simulink library "CTRL_LO_ST1_YAWTRQLGT"  (R2023b)
settings: Solver=VariableStepAuto  StartTime=0.0  StopTime=10.0  RelTol=1e-3
settings Model: Creator=blatak  LastModifiedBy=blatak

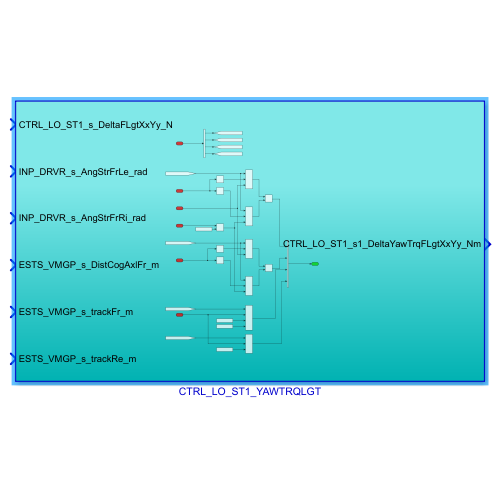
[thumbnail: Simulink's stored preview of the top-level diagram]
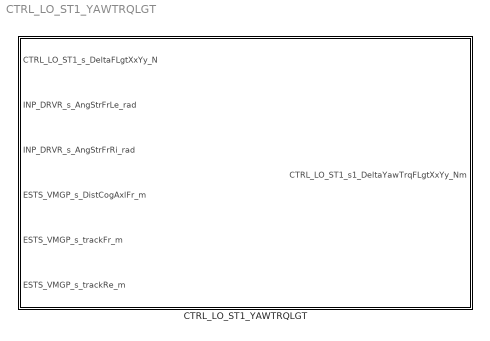
== system CTRL_LO_ST1_YAWTRQLGT ==
  CTRL_LO_ST1_YAWTRQLGT : Subsystem

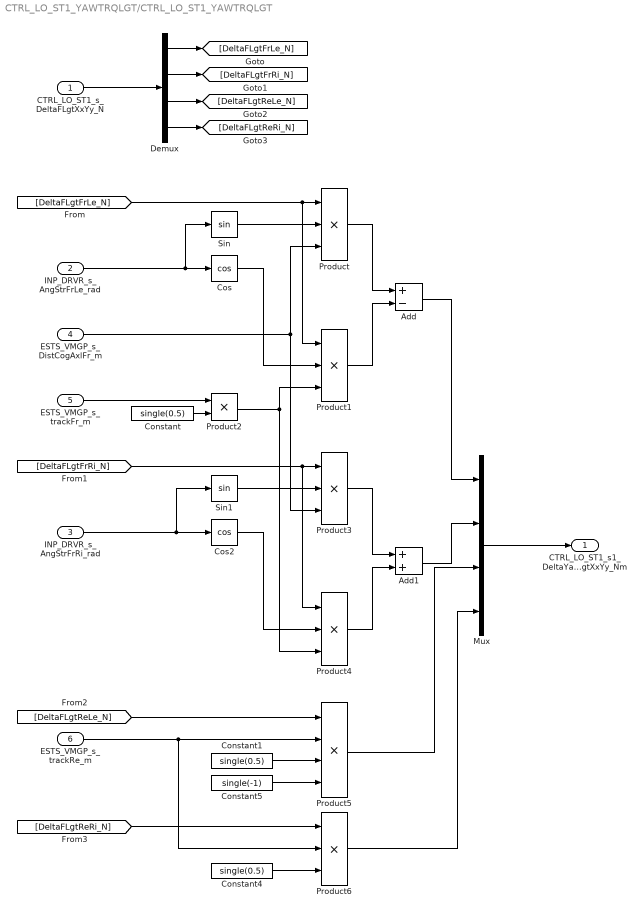
== system CTRL_LO_ST1_YAWTRQLGT/CTRL_LO_ST1_YAWTRQLGT ==
  CTRL_LO_ST1_s_DeltaFLgtXxYy_N : Inport
  INP_DRVR_s_AngStrFrLe_rad : Inport  Port=2
  INP_DRVR_s_AngStrFrRi_rad : Inport  Port=3
  ESTS_VMGP_s_DistCogAxlFr_m : Inport  Port=4
  ESTS_VMGP_s_trackFr_m : Inport  Port=5
  ESTS_VMGP_s_trackRe_m : Inport  Port=6
  Add : Sum  Inputs=+-
  Add1 : Sum
  Constant : Constant  Value=single(0.5)
  Constant1 : Constant  Value=single(0.5)
  Constant4 : Constant  Value=single(0.5)
  Constant5 : Constant  Value=single(-1)
  Cos : Trigonometry  Operator=cos
  Cos2 : Trigonometry  Operator=cos
  Demux : Demux
  Mux : Mux
  Product{,1,3..4,6} (5 alike) : Product  Inputs=3
  Product2 : Product
  Product5 : Product  Inputs=4
  Sin : Trigonometry
  Sin1 : Trigonometry
  CTRL_LO_ST1_s1_DeltaYawTrqFLgtXxYy_Nm : Outport
  wires:
  ESTS_VMGP_s_trackRe_m/1 -> Product6/2, Product5/2
  Constant/1 -> Product2/2
  Cos/1 -> Product1/2
  INP_DRVR_s_AngStrFrRi_rad/1 -> Sin1/1, Cos2/1
  Demux/3 -> [DeltaFLgtReLe_N]
  Constant5/1 -> Product5/4
  Product2/1 -> Product4/3, Product1/3
  [DeltaFLgtFrLe_N] -> Product1/1, Product/1
  ESTS_VMGP_s_DistCogAxlFr_m/1 -> Product/3, Product3/3
  Product6/1 -> Mux/4
  CTRL_LO_ST1_s_DeltaFLgtXxYy_N/1 -> Demux/1
  ESTS_VMGP_s_trackFr_m/1 -> Product2/1
  Demux/2 -> [DeltaFLgtFrRi_N]
  [DeltaFLgtReLe_N] -> Product5/1
  INP_DRVR_s_AngStrFrLe_rad/1 -> Sin/1, Cos/1
  Mux/1 -> CTRL_LO_ST1_s1_DeltaYawTrqFLgtXxYy_Nm/1
  Add1/1 -> Mux/2
  Constant1/1 -> Product5/3
  Sin1/1 -> Product3/2
  Add/1 -> Mux/1
  Cos2/1 -> Product4/2
  Product3/1 -> Add1/1
  Product4/1 -> Add1/2
  [DeltaFLgtFrRi_N] -> Product4/1, Product3/1
  Product5/1 -> Mux/3
  Sin/1 -> Product/2
  Product/1 -> Add/1
  Demux/4 -> [DeltaFLgtReRi_N]
  Product1/1 -> Add/2
  Constant4/1 -> Product6/3
  Demux/1 -> [DeltaFLgtFrLe_N]
  [DeltaFLgtReRi_N] -> Product6/1
